simulink model "Simul"  (R2021b)
settings: Solver=VariableStepAuto  StartTime=0.0  StopTime=15  RelTol=1e-3
settings Model: Creator=Alumno103  LastModifiedBy=Alumno103

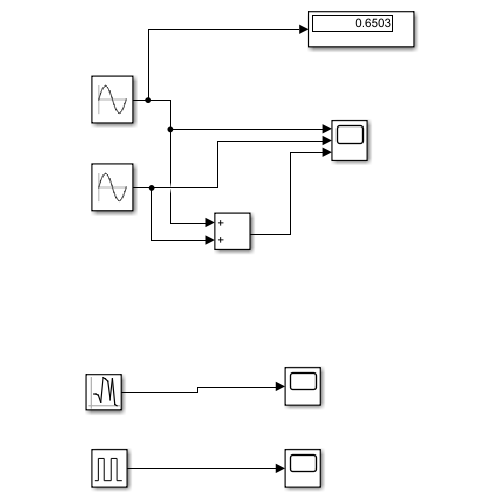
[thumbnail: Simulink's stored preview of the top-level diagram]
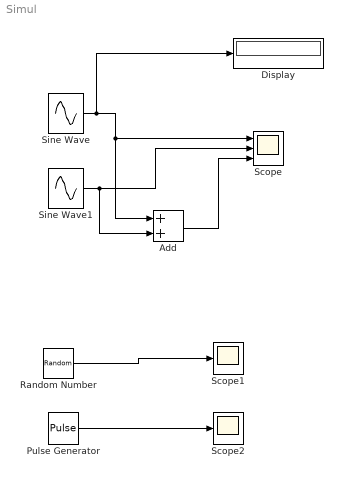
== system Simul ==
  Add : Sum
  Display : Display
  Pulse Generator : DiscretePulseGenerator  PulseType=Time based  Period=10  PulseWidth=5
  Random Number : RandomNumber  SampleTime=0.1
  Scope : Scope  NumInputPorts=3
  Scope1 : Scope
  Scope2 : Scope
  Sine Wave : Sin  SampleTime=0
  Sine Wave1 : Sin  Frequency=2  SampleTime=0
  wires:
  Sine Wave/1 -> Display/1, Add/1, Scope/1
  Sine Wave1/1 -> Add/2, Scope/2
  Add/1 -> Scope/3
  Random Number/1 -> Scope1/1
  Pulse Generator/1 -> Scope2/1
